simulink model "sim_polbereichsvorgabe_alt"  (R2016b)
settings: Solver=VariableStepAuto  StartTime=0.0  StopTime=30.0  FixedStep=1e-3  RelTol=1e3
values from neighbouring files (symbols this model uses):
  A_D = -x(8)    [calc_regler_polbereichsvorgabe.m]
  B_D = [-x(5), -x(6), -x(7)]    [calc_regler_polbereichsvorgabe.m]
  C_D = x(4)    [calc_regler_polbereichsvorgabe.m]
  D_D = [x(1), x(2), x(3)]    [calc_regler_polbereichsvorgabe.m]
  matA_g = [matA                      matE*matC_s ... (first row only)    [calcSysMatrix.m]    (also in calcSysMatrixBEO.m)
  matB = [0; (2*pi*sys.R*sys.K_K)/(sys.ue*sys.T_K); 0; (-2*pi*sys.R*sys.K_K)/(sys.ue*sys.T_K*sys.L)]    [calcSysMatrix.m]    (also in calcSysMatrixBEO.m = [0; (2*pi*sys.R*sys.K_K)/(sys.ue*sys.T_K)])
  matB_g = [matB; zeros(1,size(matB,2))]    [calcSysMatrix.m]    (also in calcSysMatrixBEO.m)
  matC_g = [matC zeros(size(matC,1),1)]    [calcSysMatrix.m]    (also in calcSysMatrixBEO.m)
  matE = matB    [calcSysMatrix.m]    (also in calcSysMatrixBEO.m)
  matR = 1    [calcKalmanKlein.m]
undefined symbols (not defined in the file or in its folder): A_b_angle, B_b_angle, C_b_angle, Continuous, D_b_angle, system, Time
libraries: simulink x5, ctrlSharedLib x1
settings Model: Creator=nicol  LastModifiedBy=nicol

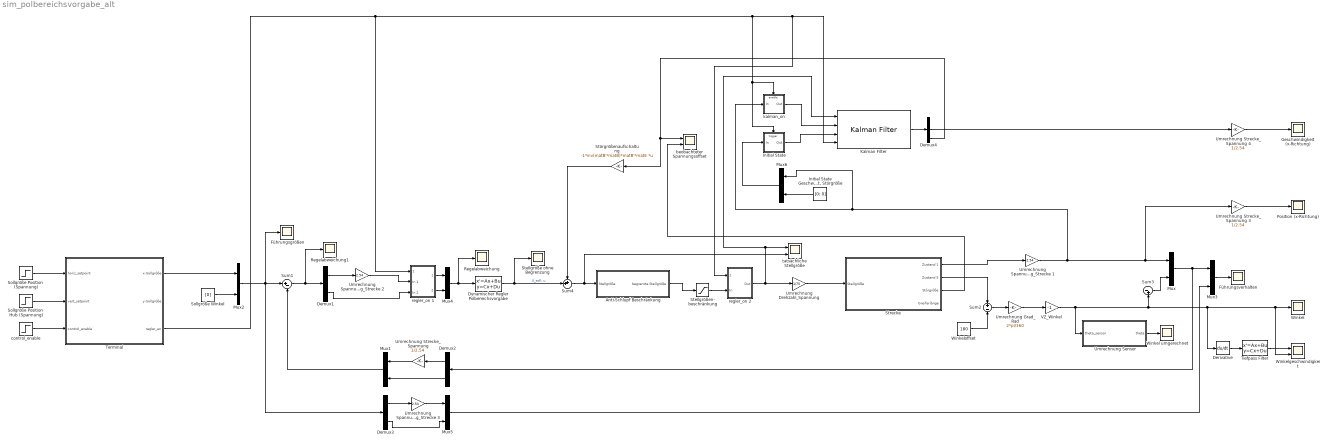
== system sim_polbereichsvorgabe_alt ==
  Anti-Schlupf Beschränkung : Subsystem
  Demux1 : Demux  Outputs=2
  Demux2 : Demux  Outputs=2
  Demux3 : Demux  Outputs=2
  Demux4 : Demux  Outputs=3
  Derivative : Derivative
  Dynamischer Regler Polbereichsvorgabe : StateSpace  A=A_D  B=-B_D  C=-C_D  D=D_D  X0=0
  Führungsgrößen : Scope
  Führungsverhalten : Scope
  Geschwindigkeit (x-Richtung) : Scope
  Initial State : Subsystem  TreatAsAtomicUnit=on
  "Initial State Geschwindigkeit, Störgröße" : Constant  Value=[0; 0]  VectorParams1D=off
  Kalman Filter : ctrlSharedLib/Kalman Filter  TimeDomain=Continuous-Time  UseCurrentEstimator=on  ModelSource=Individual A, B, C, D matrices  ModelSourceVariable=ss(0.95,1,1,0,1)  A=matA_g  B=matB_g  C=matC_g  D=0  NumberOfStates=1  NumberOfInputs=1  NumberOfOutputs=1  InitialEstimateSource=Input port  X0=0  P0=10  UseK=off  UseGH=on  NumberOfProcessNoiseInputs=1  G=matG  TimeInvariantG=on  H=0  TimeInvariantH=on  Q=matQ  TimeInvariantQ=on  R=matR  TimeInvariantR=on  N=0  TimeInvariantN=on  AddInputPort=on  AddEnablePort=off  ExternalReset=Rising  OutputEstimatedY=off  OutputP=off  Ts=-1
  Mux{,1..6} (7 alike) : Mux  Inputs=2
  Position (x-Richtung) : Scope
  Regelabweichung : Scope
  Regelabweichung1 : Scope
  Sollgröße Position (Spannung) : Step  Time=2  SampleTime=0
  Sollgröße Position Hub (Spannung) : Step  Time=2  After=0.5  SampleTime=0
  Sollgröße Winkel : Constant  Value=[0]  VectorParams1D=off
  Stellgröße ohne Begrenzung : Scope
  Stellgrößen- beschränkung : Saturate  UpperLimit=75  LowerLimit=-75
  Strecke : Subsystem
  Störgrößenaufschaltung : Gain  Gain=-1*inv(matB'*matB)*matB'*matE  Multiplication=Matrix(K*u)
  Sum1 : Sum  Inputs=|+-
  Sum2 : Sum  Inputs=+|-
  Sum3 : Sum  Inputs=|-+
  Sum4 : Sum  Inputs=++|
  Terminal : Subsystem
  Tiefpass Filter : StateSpace  A=A_b_angle  B=B_b_angle  C=C_b_angle  D=D_b_angle  X0=0
  Umrechnung Drehzahl_Spannung : Gain  Gain=1/75
  Umrechnung Grad_Rad : Gain  Gain=2*pi/360
  Umrechnung Spannung_Strecke 1 : Gain  Gain=2.54
  Umrechnung Spannung_Strecke 2 : Gain  Gain=2.54
  Umrechnung Spannung_Strecke 3 : Gain  Gain=2.54
  Umrechnung Strecke_Spannung : Gain  Gain=1/2.54
  Umrechnung Strecke_Spannung 3 : Gain  Gain=1/2.54
  Umrechnung Strecke_Spannung 4 : Gain  Gain=1/2.54
  Umrechnung Sensor : MATLAB Function  TreatAsAtomicUnit=on
  VZ_Winkel : Gain  Gain=-1
  Winkel : Scope
  Winkel umgerechnet : Scope
  Winkelgeschwindigkeit : Scope  NumInputPorts=2
  Winkeloffset : Constant  Value=180
  beobachteter Spannungsoffset : Scope  NumInputPorts=2
  control_enable : Step  Time=0  SampleTime=0
  kalman_on : Subsystem  TreatAsAtomicUnit=on
  regler_on 1 : Subsystem
  regler_on 2 : Subsystem
  tatsächliche Stellgröße : Scope  NumInputPorts=2
  wires:
  Dynamischer Regler Polbereichsvorgabe/1 -> Sum4/2, Stellgröße ohne Begrenzung/1  "U_soll; u"
  Mux/1 -> Demux2/1, Mux3/1
  Sollgröße Winkel/1 -> Mux2/2
  Mux3/1 -> Führungsverhalten/1
  Strecke/3(Störgröße) -> beobachteter Spannungsoffset/2
  Umrechnung Sensor/1(theta) -> Winkel umgerechnet/1
  Sum2/1 -> Umrechnung Grad_Rad/1
  Winkeloffset/1 -> Sum2/2
  Umrechnung Grad_Rad/1 -> VZ_Winkel/1
  VZ_Winkel/1 -> Umrechnung Sensor/1(theta_sensor), Sum3/2, Derivative/1, Winkelgeschwindigkeit/2, Winkel/1
  Anti-Schlupf Beschränkung/1(begrenzte Stellgröße) -> Stellgrößen- beschränkung/1
  Demux4/3 -> Störgrößenaufschaltung/1, beobachteter Spannungsoffset/1
  Demux2/1 -> Umrechnung Strecke_Spannung/1
  Umrechnung Strecke_Spannung/1 -> Mux1/1
  Demux2/2 -> Mux1/2
  Umrechnung Spannung_Strecke 2/1 -> regler_on 1/2(In 1)
  Demux1/1 -> Umrechnung Spannung_Strecke 2/1
  Demux1/2 -> regler_on 1/3(In 2)
  Sum1/1 -> Demux1/1, Regelabweichung1/1
  Umrechnung Spannung_Strecke 3/1 -> Mux5/1
  Demux3/1 -> Umrechnung Spannung_Strecke 3/1
  Demux3/2 -> Mux5/2
  Mux2/1 -> Sum1/1, Führungsgrößen/1, Demux3/1
  Mux5/1 -> Mux3/2
  Mux1/1 -> Sum1/2
  Terminal/3(regler_an) -> regler_on 1/1(regler_ on), regler_on 2/1(regler_ on), Kalman Filter/4, kalman_on/Enable, Initial State/Trigger
  Strecke/2(Zustand 5) -> Sum2/1
  Sum4/1 -> tatsächliche Stellgröße/2, Anti-Schlupf Beschränkung/1(Stellgröße)
  Strecke/1(Zustand 1) -> Umrechnung Spannung_Strecke 1/1
  Kalman Filter/1 -> Demux4/1
  Initial State/1(Out) -> Kalman Filter/3
  kalman_on/1(Out) -> Kalman Filter/2
  Mux6/1 -> Initial State/1(In)
  "Initial State Geschwindigkeit, Störgröße"/1 -> Mux6/2
  Umrechnung Spannung_Strecke 1/1 -> Umrechnung Strecke_Spannung 3/1, Mux/1, kalman_on/1(In), Mux6/1
  Umrechnung Drehzahl_Spannung/1 -> Strecke/1(Stellgröße)
  regler_on 1/2(Out 2) -> Mux4/2
  regler_on 1/1(Out 1) -> Mux4/1
  Mux4/1 -> Regelabweichung/1, Dynamischer Regler Polbereichsvorgabe/1
  Stellgrößen- beschränkung/1 -> regler_on 2/2(In)
  Derivative/1 -> Tiefpass Filter/1
  Tiefpass Filter/1 -> Winkelgeschwindigkeit/1
  Sollgröße Position (Spannung)/1 -> Terminal/1(horiz_setpoint)
  control_enable/1 -> Terminal/3(control_enable)
  Sollgröße Position Hub (Spannung)/1 -> Terminal/2(vert_setpoint)
  Terminal/1(x-Sollgröße) -> Mux2/1
  Störgrößenaufschaltung/1 -> Sum4/1
  Umrechnung Strecke_Spannung 3/1 -> Position (x-Richtung)/1
  Umrechnung Strecke_Spannung 4/1 -> Geschwindigkeit (x-Richtung)/1
  Demux4/2 -> Umrechnung Strecke_Spannung 4/1
  Sum3/1 -> Mux/2
  regler_on 2/1(Out) -> Umrechnung Drehzahl_Spannung/1, Kalman Filter/1, tatsächliche Stellgröße/1

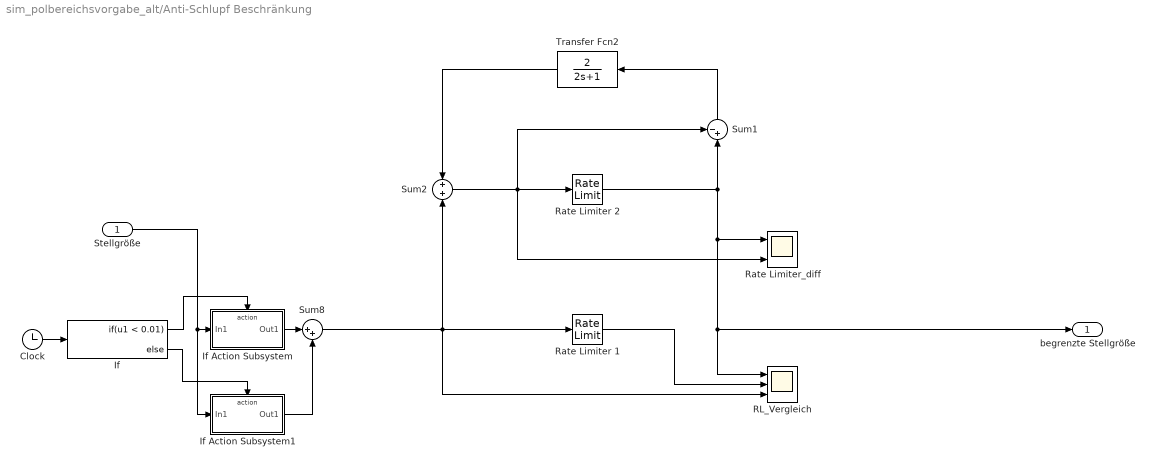
== system sim_polbereichsvorgabe_alt/Anti-Schlupf Beschränkung ==
  Stellgröße : Inport
  Clock : Clock
  If : If  IfExpression=u1 < 0.01
  If Action Subsystem : Subsystem  TreatAsAtomicUnit=on
  If Action Subsystem1 : Subsystem  TreatAsAtomicUnit=on
  RL_Vergleich : Scope  NumInputPorts=3
  Rate Limiter 1 : RateLimiter  RisingSlewLimit=9.57  FallingSlewLimit=-9.57  SampleTimeMode=inherited
  Rate Limiter 2 : RateLimiter  RisingSlewLimit=9.57  FallingSlewLimit=-9.57  SampleTimeMode=inherited
  Rate Limiter_diff : Scope  NumInputPorts=2
  Sum1 : Sum  Inputs=-+|
  Sum2 : Sum  Inputs=+|+
  Sum8 : Sum  Inputs=|++
  Transfer Fcn2 : TransferFcn  Numerator=[2]  Denominator=[2 1]
  begrenzte Stellgröße : Outport
  wires:
  Stellgröße/1 -> If Action Subsystem1/1(In1), If Action Subsystem/1(In1)
  If Action Subsystem/1(Out1) -> Sum8/1
  If Action Subsystem1/1(Out1) -> Sum8/2
  Clock/1 -> If/1
  If/1 -> If Action Subsystem/Action
  If/2 -> If Action Subsystem1/Action
  Sum8/1 -> RL_Vergleich/3, Sum2/2, Rate Limiter 1/1
  Sum2/1 -> Rate Limiter_diff/2, Sum1/1, Rate Limiter 2/1
  Sum1/1 -> Transfer Fcn2/1
  Transfer Fcn2/1 -> Sum2/1
  Rate Limiter 2/1 -> begrenzte Stellgröße/1, RL_Vergleich/1, Rate Limiter_diff/1, Sum1/2
  Rate Limiter 1/1 -> RL_Vergleich/2

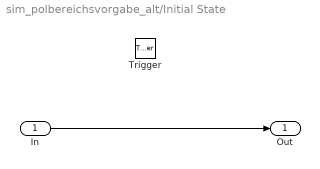
== system sim_polbereichsvorgabe_alt/Initial State ==
  In : Inport
  Trigger : TriggerPort  VariantControl=Variant
  Out : Outport
  wires:
  In/1 -> Out/1

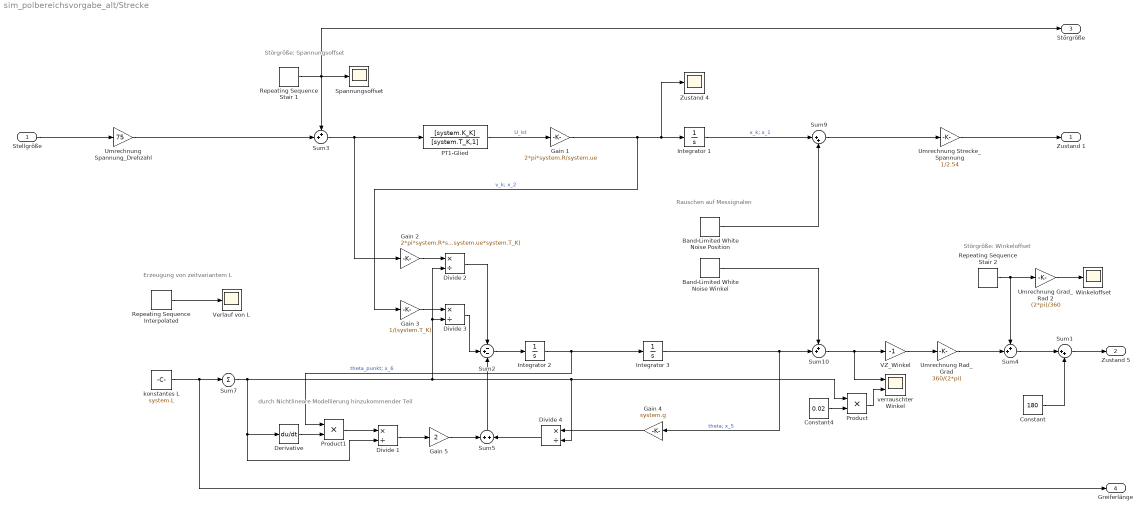
== system sim_polbereichsvorgabe_alt/Strecke ==
  note: Störgröße: Spannungsoffset
  note: durch Nichtlineare Modellierung hinzukommender Teil
  note: Rauschen auf Messignalen
  note: Erzeugung von zeitvariantem L
  note: Störgröße: Winkeloffset
  Stellgröße : Inport
  Band-Limited White Noise Position : simulink/Sources/Band-Limited White Noise  Cov=[0.0000001]  Ts=0.01  seed=[23341]
  Band-Limited White Noise Winkel : simulink/Sources/Band-Limited White Noise  Cov=[0.000000001]  Ts=0.01  seed=[23341]
  Constant : Constant  Value=180
  Constant4 : Constant  Value=0.02
  Derivative : Derivative
  Divide {1..4} (4 alike) : Product  Inputs=*/
  Gain 1 : Gain  Gain=2*pi*system.R/system.ue
  Gain 2 : Gain  Gain=2*pi*system.R*system.K_K/(system.ue*system.T_K)
  Gain 3 : Gain  Gain=1/(system.T_K)
  Gain 4 : Gain  Gain=system.g
  Gain 5 : Gain  Gain=2
  Integrator 1 : Integrator
  Integrator 2 : Integrator
  Integrator 3 : Integrator
  PT1-Glied : TransferFcn  Numerator=[system.K_K]  Denominator=[system.T_K,1]
  Product : Product
  Product1 : Product
  Repeating Sequence Interpolated : simulink/Sources/Repeating Sequence Interpolated  OutValues=[1.5 1.0 0.7 0.5 0.4 0.3 0.2 0.5 1.5 1.0 0.2 0.2 1.0 1.5 0.5 0.2].'  TimeValues=[0 2 4 6 8 10 12 14 16 18 20 22 24 26 28 30].'  LookUpMeth=Interpolation-Use End Values  tsamp=0.001  OutMin=[]  OutMax=[]  OutDataTypeStr=double  OutputDataTypeScalingMode=double  OutDataType=fixdt(0,8)  OutScaling=2^-10
  Repeating Sequence Stair 1 : simulink/Sources/Repeating Sequence Stair  OutValues=[0.05 0.05 0.05 0.05 0.05].'  tsamp=5  OutMin=[]  OutMax=[]  OutDataTypeStr=double  OutputDataTypeScalingMode=double  OutDataType=fixdt(0,8)  ConRadixGroup=Best Precision: Vector-wise  OutScaling=2^-12
  Repeating Sequence Stair 2 : simulink/Sources/Repeating Sequence Stair  OutValues=[10 10 10 10 10 10].'  tsamp=5  OutMin=[]  OutMax=[]  OutDataTypeStr=double  OutputDataTypeScalingMode=double  OutDataType=fixdt(0,8)  ConRadixGroup=Best Precision: Vector-wise  OutScaling=2^-12
  Spannungsoffset : Scope
  Sum1 : Sum  Inputs=|++
  Sum10 : Sum  Inputs=++|
  Sum2 : Sum  Inputs=-+-
  Sum3 : Sum  Inputs=++|
  Sum4 : Sum  Inputs=++|
  Sum5 : Sum  Inputs=+|+
  Sum7 : Sum  Inputs=|+|
  Sum9 : Sum  Inputs=|++
  Umrechnung Grad_Rad 2 : Gain  Gain=(2*pi)/360
  Umrechnung Rad_Grad : Gain  Gain=360/(2*pi)
  Umrechnung Spannung_Drehzahl : Gain  Gain=75
  Umrechnung Strecke_Spannung : Gain  Gain=1/2.54
  VZ_Winkel : Gain  Gain=-1
  Verlauf von L : Scope
  Winkeloffset : Scope
  Zustand 4 : Scope
  konstantes L : Constant  Value=system.L
  verrauschter Winkel : Scope  NumInputPorts=2
  Zustand 1 : Outport
  Zustand 5 : Outport  Port=2
  Störgröße : Outport  Port=3
  Greiferlänge : Outport  Port=4
  wires:
  PT1-Glied/1 -> Gain 1/1  "U_ist"
  Gain 1/1 -> Zustand 4/1, Integrator 1/1, Gain 3/1  "v_k; x_2"
  Sum2/1 -> Integrator 2/1
  Integrator 2/1 -> Product1/1, Integrator 3/1  "theta_punkt; x_6"
  Sum3/1 -> PT1-Glied/1, Gain 2/1
  Repeating Sequence Stair 1/1 -> Sum3/1, Störgröße/1, Spannungsoffset/1
  Repeating Sequence Interpolated/1 -> Verlauf von L/1
  Gain 2/1 -> Divide 2/1
  Divide 2/1 -> Sum2/1
  Gain 3/1 -> Divide 3/1
  Divide 3/1 -> Sum2/2
  Gain 4/1 -> Divide 4/1
  Product/1 -> verrauschter Winkel/2
  Constant4/1 -> Product/2
  Integrator 1/1 -> Sum9/1  "x_k; x_1"
  Sum9/1 -> Umrechnung Strecke_Spannung/1
  Divide 4/1 -> Sum5/2
  Sum5/1 -> Sum2/3
  Gain 5/1 -> Sum5/1
  Product1/1 -> Divide 1/1
  Divide 1/1 -> Gain 5/1
  Derivative/1 -> Product1/2
  Stellgröße/1 -> Umrechnung Spannung_Drehzahl/1
  Umrechnung Spannung_Drehzahl/1 -> Sum3/2
  Umrechnung Strecke_Spannung/1 -> Zustand 1/1
  Sum10/1 -> VZ_Winkel/1, verrauschter Winkel/1
  Sum1/1 -> Zustand 5/1
  Constant/1 -> Sum1/2
  VZ_Winkel/1 -> Umrechnung Rad_Grad/1
  Band-Limited White Noise Position/1 -> Sum9/2
  Band-Limited White Noise Winkel/1 -> Sum10/1
  Repeating Sequence Stair 2/1 -> Umrechnung Grad_Rad 2/1, Sum4/1
  Integrator 3/1 -> Gain 4/1, Sum10/2  "theta; x_5"
  Sum7/1 -> Divide 1/2, Derivative/1, Divide 3/2, Divide 2/2, Divide 4/2, Product/1
  Sum4/1 -> Sum1/1
  Umrechnung Rad_Grad/1 -> Sum4/2
  Umrechnung Grad_Rad 2/1 -> Winkeloffset/1
  konstantes L/1 -> Greiferlänge/1, Sum7/1

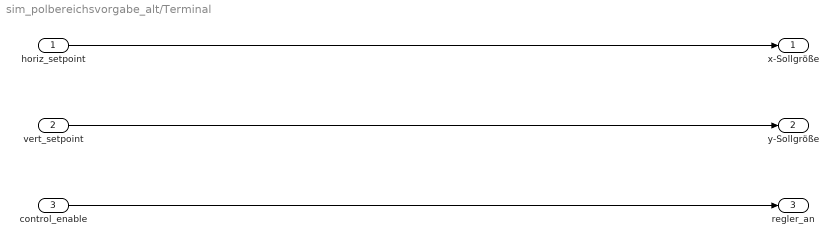
== system sim_polbereichsvorgabe_alt/Terminal ==
  horiz_setpoint : Inport
  vert_setpoint : Inport  Port=2
  control_enable : Inport  Port=3
  x-Sollgröße : Outport
  y-Sollgröße : Outport  Port=2
  regler_an : Outport  Port=3
  wires:
  horiz_setpoint/1 -> x-Sollgröße/1
  vert_setpoint/1 -> y-Sollgröße/1
  control_enable/1 -> regler_an/1

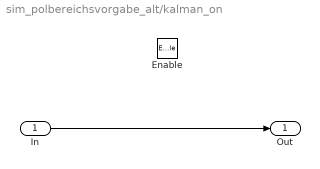
== system sim_polbereichsvorgabe_alt/kalman_on ==
  In : Inport
  Enable : EnablePort
  Out : Outport
  wires:
  In/1 -> Out/1

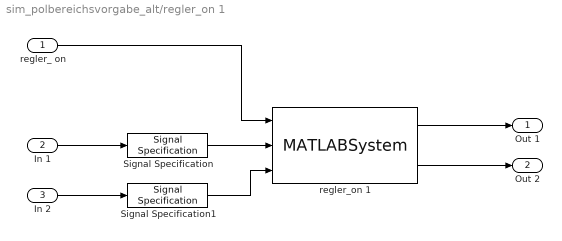
== system sim_polbereichsvorgabe_alt/regler_on 1 ==
  regler_ on : Inport
  In 1 : Inport  Port=2
  In 2 : Inport  Port=3
  Signal Specification : SignalSpecification  Dimensions=1
  Signal Specification1 : SignalSpecification  Dimensions=1
  regler_on 1 : MATLABSystem  System=regler_switch_2  SimulateUsing=Code generation
      mask Type: regler_switch_2
      mask Display:
      | disp('regler_switch_2');
      | port_label('input',1,'regler_on');
      | port_label('input',2,'input1');
      | port_label('input',3,'input2');
      | port_label('output',1,'y1');
      | port_label('output',2,'y2');
  Out 1 : Outport
  Out 2 : Outport  Port=2
  wires:
  regler_on 1/1 -> Out 1/1
  regler_on 1/2 -> Out 2/1
  In 2/1 -> Signal Specification1/1
  In 1/1 -> Signal Specification/1
  Signal Specification/1 -> regler_on 1/2
  Signal Specification1/1 -> regler_on 1/3
  regler_ on/1 -> regler_on 1/1

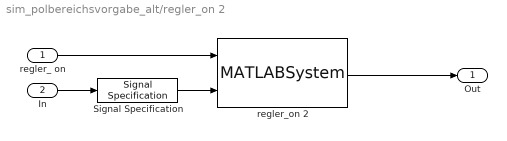
== system sim_polbereichsvorgabe_alt/regler_on 2 ==
  regler_ on : Inport
  In : Inport  Port=2
  Signal Specification : SignalSpecification  Dimensions=1
  regler_on 2 : MATLABSystem  System=regler_switch_1  SimulateUsing=Code generation
      mask Type: regler_switch_1
      mask Display:
      | disp('regler_switch_1');
      | port_label('input',1,'regler_on');
      | port_label('input',2,'input');
      | port_label('output',1,'y');
  Out : Outport
  wires:
  regler_ on/1 -> regler_on 2/1
  regler_on 2/1 -> Out/1
  Signal Specification/1 -> regler_on 2/2
  In/1 -> Signal Specification/1

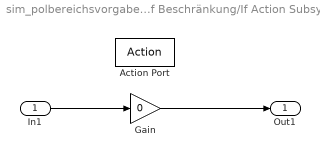
== system sim_polbereichsvorgabe_alt/Anti-Schlupf Beschränkung/If Action Subsystem ==
  In1 : Inport
  Action Port : ActionPort  ActionType=then
  Gain : Gain  Gain=0
  Out1 : Outport
  wires:
  In1/1 -> Gain/1
  Gain/1 -> Out1/1

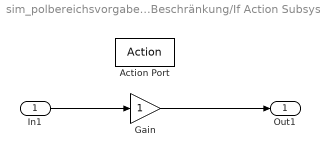
== system sim_polbereichsvorgabe_alt/Anti-Schlupf Beschränkung/If Action Subsystem1 ==
  In1 : Inport
  Action Port : ActionPort  ActionType=else
  Gain : Gain
  Out1 : Outport
  wires:
  In1/1 -> Gain/1
  Gain/1 -> Out1/1

== matlab function sim_polbereichsvorgabe_alt/Umrechnung Sensor ==
  data: theta_sensor input; theta output
function theta  = sensorWinkel(theta_sensor)
% berechnet aus dem gemessenen Winkel den tatsächlichen Winkel des
% Lasthebers

% l_verb: Länge des Verbindungsstücks
% l_welle: Abstand der beiden Wellen

% Parameter für die Winkelumrechnung
l_verb = 0.109; % m %
l_welle = 0.0575; % m %

theta = asin(sin(theta_sensor) * (l_verb / sqrt(l_welle^2 + l_verb^2 - (2 * l_verb * l_welle * cos(theta_sensor)))));
